simulink model "DYNctl_ver4_etud_obfusc"  (R2018b)
settings: Solver=ode45  StartTime=0.0  StopTime=tfin  FixedStep=0.001  RelTol=1e-9  AbsTol=1e-12  EnableMultiTasking=on
values from neighbouring files (symbols this model uses):
  denCompAngles = 1.0e07*[0.000000100000000 0.000823402569667 1.694979479335234 0]    [run_bancessai.m]
  denCompz = 1.0e05*[0.000010000000000 0.017380342819025 5.055406372627656 0]    [run_bancessai.m]
  g = sqrt(1+yp.^2)    [Trajectoire_func.m]
  numCompAngles = 1.0e09*[0.000230814504577 0.026170635469275 0.897433010674818 9.699372248008062]    [run_bancessai.m]
  numCompz = 1.0e11*[0.000031609546854 0.004304100455063 0.142047621936623 1.354942422178642]    [run_bancessai.m]
  TABC = [YA YB YC ... (first row only)    [run_bancessai.m]
  Tdef = [YD -XD 1 ... (first row only)    [run_bancessai.m]
undefined symbols (not defined in the file or in its folder): ae0, ae1, ae2, ae3, as0, as1, as2, as3, be1, JS, Jx, Jy, L, mS, mSg, mtot, R, rS, Vmax, XA, XB, XC, XD, XE, XF, YA, YB, YC, YD, YE, YF
settings Model: Creator=delafontaine  LastModifiedBy=natgo
settings SolverCC: AlgebraicLoopSolver=LineSearch
settings DataIOCC: LimitDataPoints=on  SaveFormat=Array  SignalLoggingSaveFormat=ModelDataLogs
settings OptimizationCC: LifeSpan=inf
settings DebuggingCC: UnderspecifiedInitializationDetection=Classic  MergeDetectMultiDrivingBlocksExec=none  MultiTaskDSMMsg=warning  MultiTaskCondExecSysMsg=none  SFUnexpectedBacktrackingDiag=warning  SFNoUnconditionalDefaultTransitionDiag=warning  SFExecutionAtInitializationDiag=none
settings HardwareCC: ProdBitPerPointer=32  ProdBitPerSizeT=32  ProdBitPerPtrDiffT=32  ProdLargestAtomicFloat=None  ProdIntDivRoundTo=Undefined  ProdEndianess=Unspecified  ProdWordSize=32  ProdHWDeviceType=32-bit Generic
settings ModelReferenceCC: PropagateSignalLabelsOutOfModel=off
settings SFSimCC: SimUseLocalCustomCode=off
settings RTWCC: RTWUseLocalCustomCode=off
settings CodeAppCC: StateflowObjectComments=on
settings GRTTargetCC: TargetLangStandard=C89/C90 (ANSI)  GeneratePreprocessorConditionals=Disable all
settings ConfigComp: CovMetricSettings=dw  CovHtmlReporting=on  CovSaveCumulativeToWorkspaceVar=on  CovSaveSingleToWorkspaceVar=on  CovExternalEMLEnable=off  CovSFcnEnable=off

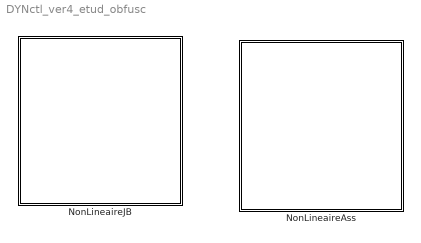
== system DYNctl_ver4_etud_obfusc ==
  NonLineaireAss : Subsystem
  NonLineaireJB : Subsystem

== system DYNctl_ver4_etud_obfusc/NonLineaireAss ==
  Asservissement 2 : Subsystem
  From Workspace1 : FromWorkspace  VariableName=z_des  SampleTime=0  Interpolate=off  OutputAfterFinalValue=Holding final value
  From Workspace4 : FromWorkspace  VariableName=x_des  SampleTime=0  Interpolate=off  OutputAfterFinalValue=Holding final value
  From Workspace6 : FromWorkspace  VariableName=y_des  SampleTime=0  Interpolate=off  OutputAfterFinalValue=Holding final value
  Mux1 : Mux  Inputs=25
  Systeme non lineaire : Subsystem
  To Workspace2 : ToWorkspace  VariableName=ySystemeNonLineaire  SampleTime=-1
  To Workspace6 : ToWorkspace  VariableName=Ax_des1  SampleTime=-1
  To Workspace7 : ToWorkspace  VariableName=Ay_des1  SampleTime=-1
  wires:
  Systeme non lineaire/6(Ib) -> Mux1/6
  Systeme non lineaire/21(zB) -> Mux1/21
  Systeme non lineaire/12(Wx) -> Mux1/12
  Asservissement 2/5(Vc) -> Systeme non lineaire/3(Vc)
  Asservissement 2/3(Va) -> Systeme non lineaire/1(Va)
  Asservissement 2/4(Vb) -> Systeme non lineaire/2(Vb)
  Systeme non lineaire/3(Vy) -> Asservissement 2/6(Vy), Mux1/3
  Systeme non lineaire/17(VA) -> Mux1/17
  Systeme non lineaire/23(zD) -> Asservissement 2/7(zD), Mux1/23
  Asservissement 2/1(Axcalcule) -> To Workspace6/1, Asservissement 2/11(Aydes)
  Systeme non lineaire/5(Ia) -> Mux1/5
  Systeme non lineaire/4(Vx) -> Asservissement 2/3(Vx), Mux1/4
  Systeme non lineaire/8(Ay) -> Mux1/8
  Systeme non lineaire/2(x) -> Asservissement 2/2(Px), Mux1/2
  Systeme non lineaire/9(Ax) -> Mux1/9
  Systeme non lineaire/15(Fb) -> Mux1/15
  Systeme non lineaire/16(Fc) -> Mux1/16
  Systeme non lineaire/1(y) -> Asservissement 2/5(Py), Mux1/1
  Systeme non lineaire/11(Vz) -> Mux1/11
  From Workspace4/1 -> Asservissement 2/1(xdes)
  Mux1/1 -> To Workspace2/1
  Systeme non lineaire/19(VC) -> Mux1/19
  Systeme non lineaire/13(Wy) -> Mux1/13
  Systeme non lineaire/7(Ic) -> Mux1/7
  Systeme non lineaire/10(Pz) -> Mux1/10
  Systeme non lineaire/22(zC) -> Mux1/22
  Asservissement 2/2(Aycalcule) -> To Workspace7/1, Asservissement 2/10(Axdes)
  Systeme non lineaire/25(zF) -> Asservissement 2/9(zF), Mux1/25
  Systeme non lineaire/20(zA) -> Mux1/20
  Systeme non lineaire/24(zE) -> Asservissement 2/8(zE), Mux1/24
  Systeme non lineaire/18(VB) -> Mux1/18
  Systeme non lineaire/14(Fa) -> Mux1/14
  From Workspace6/1 -> Asservissement 2/4(ydes)
  From Workspace1/1 -> Asservissement 2/12(zdes)

== system DYNctl_ver4_etud_obfusc/NonLineaireJB ==
  Asservissements : Subsystem
      mask help: Simulink:masks:GenSFuncDesc_MD
      mask Help: eval('feval(''rtwprivate'',''rtwhelpview'',''rtw_sfcn_block'')');
  Clock : Clock
  From Workspace2 : FromWorkspace  VariableName=x_des  SampleTime=0  Interpolate=off  OutputAfterFinalValue=Holding final value
  From Workspace3 : FromWorkspace  VariableName=y_des  SampleTime=0  Interpolate=off  OutputAfterFinalValue=Holding final value
  From Workspace5 : FromWorkspace  VariableName=z_des  SampleTime=0  Interpolate=off  OutputAfterFinalValue=Holding final value
  ModeleNonLineaire : Subsystem
      mask help: Simulink:masks:GenSFuncDesc_MD
      mask Help: eval('feval(''rtwprivate'',''rtwhelpview'',''rtw_sfcn_block'')');
  Mux : Mux  Inputs=25
  To Workspace : ToWorkspace  VariableName=tsim  SampleTime=-1
  To Workspace1 : ToWorkspace  VariableName=ynonlineaire  SampleTime=-1
  To Workspace10 : ToWorkspace  VariableName=z_des_out  SampleTime=-1
  To Workspace6 : ToWorkspace  VariableName=Ax_des  SampleTime=-1
  To Workspace7 : ToWorkspace  VariableName=Ay_des  SampleTime=-1
  To Workspace8 : ToWorkspace  VariableName=y_des_out  SampleTime=-1
  To Workspace9 : ToWorkspace  VariableName=x_des_out  SampleTime=-1
  wires:
  ModeleNonLineaire/7(Px) -> Asservissements/9(Px), Mux/7  "Px"
  ModeleNonLineaire/5(Wy) -> Mux/5  "Wy"
  From Workspace5/1 -> Asservissements/6(zdes), To Workspace10/1
  ModeleNonLineaire/18(zE) -> Asservissements/2(zE), Mux/18
  ModeleNonLineaire/1(Ax) -> Mux/1  "Ax"
  Asservissements/4(Axcalcule) -> Asservissements/4(Axdes), To Workspace6/1
  ModeleNonLineaire/11(IA) -> Mux/11  "IA"
  Clock/1 -> To Workspace/1
  ModeleNonLineaire/2(Ay) -> Mux/2  "Ay"
  Asservissements/5(Aycalcule) -> Asservissements/5(Aydes), To Workspace7/1
  ModeleNonLineaire/19(zF) -> Asservissements/3(zF), Mux/19
  Mux/1 -> To Workspace1/1
  ModeleNonLineaire/12(IB) -> Mux/12  "IB"
  ModeleNonLineaire/3(Pz) -> Mux/3  "Pz"
  ModeleNonLineaire/21(FB) -> Mux/21
  ModeleNonLineaire/17(zD) -> Asservissements/1(zD), Mux/17
  ModeleNonLineaire/24(VB) -> Mux/24
  ModeleNonLineaire/14(zA) -> Mux/14
  ModeleNonLineaire/9(Vx) -> Asservissements/11(Vx), Mux/9  "Vx"
  From Workspace2/1 -> Asservissements/7(xdes), To Workspace9/1
  ModeleNonLineaire/4(Wx) -> Mux/4  "Wx"
  ModeleNonLineaire/10(Vy) -> Asservissements/12(Vy), Mux/10  "Vy"
  ModeleNonLineaire/16(zC) -> Mux/16
  ModeleNonLineaire/15(zB) -> Mux/15
  ModeleNonLineaire/13(IC) -> Mux/13  "IC"
  ModeleNonLineaire/8(Py) -> Asservissements/10(Py), Mux/8  "Py"
  From Workspace3/1 -> Asservissements/8(ydes), To Workspace8/1
  ModeleNonLineaire/6(Vz) -> Mux/6  "Vz"
  ModeleNonLineaire/25(VC) -> Mux/25
  Asservissements/1(VAcalcule) -> ModeleNonLineaire/1(VAdesire)
  ModeleNonLineaire/22(FC) -> Mux/22
  Asservissements/3(VCcalcule) -> ModeleNonLineaire/3(VCdesire)
  ModeleNonLineaire/20(FA) -> Mux/20
  ModeleNonLineaire/23(VA) -> Mux/23
  Asservissements/2(VBcalcule) -> ModeleNonLineaire/2(VBdesire)

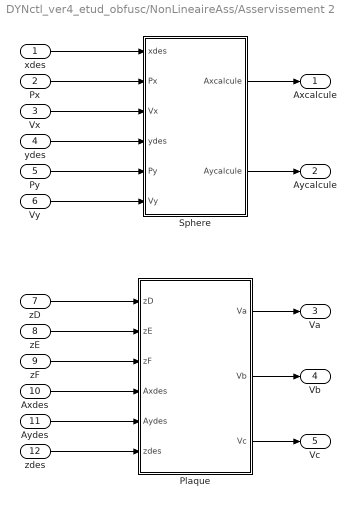
== system DYNctl_ver4_etud_obfusc/NonLineaireAss/Asservissement 2 ==
  xdes : Inport
  Px : Inport  Port=2
  Vx : Inport  Port=3
  ydes : Inport  Port=4
  Py : Inport  Port=5
  Vy : Inport  Port=6
  zD : Inport  Port=7
  zE : Inport  Port=8
  zF : Inport  Port=9
  Axdes : Inport  Port=10
  Aydes : Inport  Port=11
  zdes : Inport  Port=12
  Plaque : Subsystem
  Sphere : Subsystem
  Axcalcule : Outport
  Aycalcule : Outport  Port=2
  Va : Outport  Port=3
  Vb : Outport  Port=4
  Vc : Outport  Port=5
  wires:
  xdes/1 -> Sphere/1(xdes)
  Px/1 -> Sphere/2(Px)
  Vx/1 -> Sphere/3(Vx)
  ydes/1 -> Sphere/4(ydes)
  Py/1 -> Sphere/5(Py)
  Vy/1 -> Sphere/6(Vy)
  Sphere/1(Axcalcule) -> Axcalcule/1
  Sphere/2(Aycalcule) -> Aycalcule/1
  zD/1 -> Plaque/1(zD)
  zE/1 -> Plaque/2(zE)
  zF/1 -> Plaque/3(zF)
  Axdes/1 -> Plaque/4(Axdes)
  Aydes/1 -> Plaque/5(Aydes)
  zdes/1 -> Plaque/6(zdes)
  Plaque/1(Va) -> Va/1
  Plaque/2(Vb) -> Vb/1
  Plaque/3(Vc) -> Vc/1

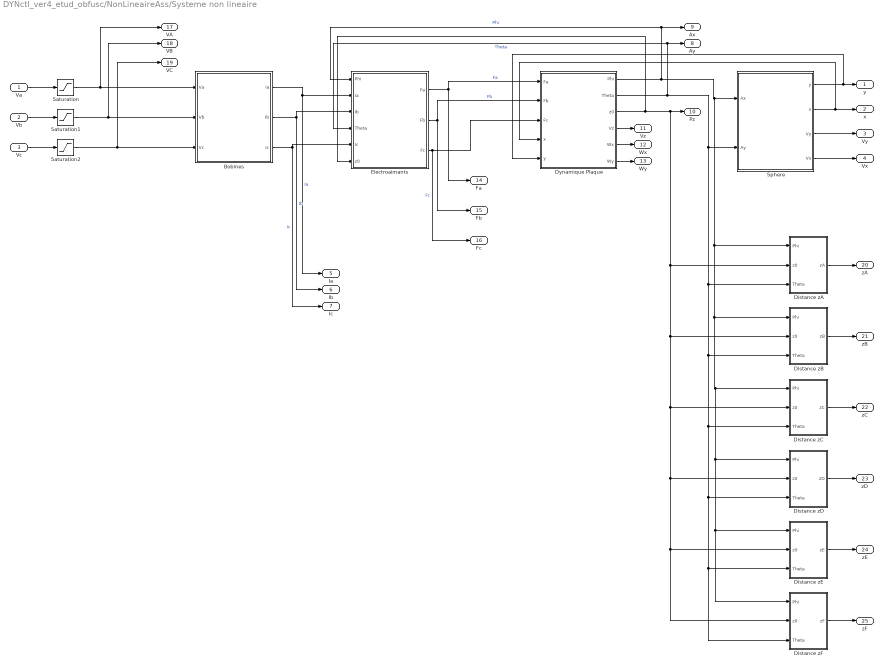
== system DYNctl_ver4_etud_obfusc/NonLineaireAss/Systeme non lineaire ==
  Va : Inport
  Vb : Inport  Port=2
  Vc : Inport  Port=3
  Bobines : Subsystem
  Distance zA : Subsystem
  Distance zB : Subsystem
  Distance zC : Subsystem
  Distance zD : Subsystem
  Distance zE : Subsystem
  Distance zF : Subsystem
  Dynamique Plaque : Subsystem
  Electroaimants : Subsystem
  Saturation : Saturate  UpperLimit=Vmax  LowerLimit=-Vmax
  Saturation1 : Saturate  UpperLimit=Vmax  LowerLimit=-Vmax
  Saturation2 : Saturate  UpperLimit=Vmax  LowerLimit=-Vmax
  Sphere : Subsystem
  y : Outport
  x : Outport  Port=2
  Vy : Outport  Port=3
  Vx : Outport  Port=4
  Ia : Outport  Port=5
  Ib : Outport  Port=6
  Ic : Outport  Port=7
  Ay : Outport  Port=8
  Ax : Outport  Port=9
  Pz : Outport  Port=10
  Vz : Outport  Port=11
  Wx : Outport  Port=12
  Wy : Outport  Port=13
  Fa : Outport  Port=14
  Fb : Outport  Port=15
  Fc : Outport  Port=16
  VA : Outport  Port=17
  VB : Outport  Port=18
  VC : Outport  Port=19
  zA : Outport  Port=20
  zB : Outport  Port=21
  zC : Outport  Port=22
  zD : Outport  Port=23
  zE : Outport  Port=24
  zF : Outport  Port=25
  wires:
  Bobines/2(Ib) -> Ib/1, Electroaimants/3(Ib)  "Ib"
  Bobines/1(Ia) -> Electroaimants/2(Ia), Ia/1  "Ia"
  Vb/1 -> Saturation1/1
  Va/1 -> Saturation/1
  Bobines/3(Ic) -> Ic/1, Electroaimants/5(Ic)  "Ic"
  Vc/1 -> Saturation2/1
  Sphere/1(y) -> y/1, Dynamique Plaque/5(y)
  Sphere/2(x) -> Dynamique Plaque/4(x), x/1
  Sphere/3(Vy) -> Vy/1
  Sphere/4(Vx) -> Vx/1
  Dynamique Plaque/4(Vz) -> Vz/1
  Dynamique Plaque/5(Wx) -> Wx/1
  Dynamique Plaque/6(Wy) -> Wy/1
  Saturation/1 -> Bobines/1(Va), VA/1
  Saturation2/1 -> Bobines/3(Vc), VC/1
  Saturation1/1 -> Bobines/2(Vb), VB/1
  Dynamique Plaque/3(z0) -> Distance zB/2(z0), Distance zF/2(z0), Distance zE/2(z0), Distance zD/2(z0), Distance zC/2(z0), Distance zA/2(z0), Pz/1, Electroaimants/6(z0)
  Distance zA/1(zA) -> zA/1
  Distance zB/1(zB) -> zB/1
  Distance zC/1(zC) -> zC/1
  Distance zD/1(zD) -> zD/1
  Distance zE/1(zE) -> zE/1
  Distance zF/1(zF) -> zF/1
  Electroaimants/1(Fa) -> Dynamique Plaque/1(Fa), Fa/1  "Fa"
  Electroaimants/2(Fb) -> Dynamique Plaque/2(Fb), Fb/1  "Fb"
  Electroaimants/3(Fc) -> Fc/1, Dynamique Plaque/3(Fc)  "Fc"
  Dynamique Plaque/1(Phi) -> Ax/1, Electroaimants/1(Phi), Distance zA/1(Phi), Distance zD/1(Phi), Distance zF/1(Phi), Distance zE/1(Phi), Distance zC/1(Phi), Distance zB/1(Phi), Sphere/1(Ax)  "Phi"
  Dynamique Plaque/2(Theta) -> Electroaimants/4(Theta), Ay/1, Distance zF/3(Theta), Distance zE/3(Theta), Distance zD/3(Theta), Distance zC/3(Theta), Distance zB/3(Theta), Distance zA/3(Theta), Sphere/2(Ay)  "Theta"

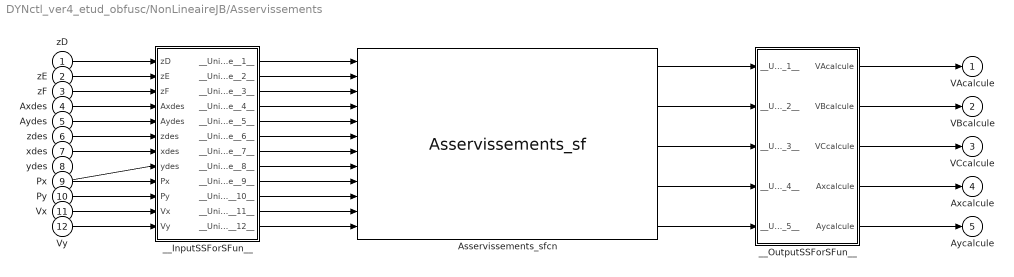
== system DYNctl_ver4_etud_obfusc/NonLineaireJB/Asservissements ==
  zD : Inport
  zE : Inport  Port=2
  zF : Inport  Port=3
  Axdes : Inport  Port=4
  Aydes : Inport  Port=5
  zdes : Inport  Port=6
  xdes : Inport  Port=7
  ydes : Inport  Port=8
  Px : Inport  Port=9
  Py : Inport  Port=10
  Vx : Inport  Port=11
  Vy : Inport  Port=12
  Asservissements_sfcn : S-Function  FunctionName=Asservissements_sf  SFunctionModules=""  SFunctionDeploymentMode=off  EnableBusSupport=off  mask{rtw_sf_name=Asservissements_sf, showVar=off}
      mask prompts: rtw_sf_name "Simulink:masks:GenSFuncName_MP"; showVar "Simulink:masks:GenSFuncShowModuleList_MP"
      mask help: Simulink:masks:GenSFuncDesc_MD
      mask init:
      | displist = '';
      | if ~strcmp(get_param(gcb, 'FunctionName'), rtw_sf_name);
      |   set_param(gcb, 'FunctionName', rtw_sf_name);
      | end
      | % Check if we are generating code
      | rtw_mode = false;
      | if strcmpi(get_param(bdroot(gcb),'SimulationStatus'),'Initializing')
      | 	rtw_mode = strcmpi(get_param(bdroot(gcb),'BuildingRTWCode'),'on') && ...
      | 		~strcmpi(get_param(bdroot(gcb),'TargetStyle'),'SimulationTarget');
      | end
      | if showVar || rtw_mode
      | 	if exist('rtwsfunc') == 2 | exist('rtwsfunc') == 6
      | 		tmplist = rtwsfunc(rtw_sf_name,gcb);
      | 		tmplist = DAStudio.message('Simulink:masks:GenSFuncListOfModules_IC', tmplist);
      | 	elseif showVar
      | 		tmplist1 = DAStudio.message('Simulink:masks:GenSFuncListOfModules_IC', '');
      |         tmplist2 = DAStudio.message('Simulink:masks:GenSFuncNotLicensed_IC');
      |         tmplist = [tmplist1 tmplist2];
      |  	end
      | end
      | if showVar
      |   displist = tmplist;
      | end
      settings: CopyFcn=|
      | if ~strcmp(get_param(gcb,'Linkstatus'),'none') && ...
      | ~strcmp(get_param(gcb,'Linkstatus'),'implicit')
      |   set_param(gcb,'LinkStatus','none');
      | end
      mask Help: eval('feval(''rtwprivate'',''rtwhelpview'',''rtw_sfcn_block'')');
      mask Display:
      | port_label('input',1,'zD');
      | port_label('input',2,'zE');
      | port_label('input',3,'zF');
      | port_label('input',4,'Axdes');
      | port_label('input',5,'Aydes');
      | port_label('input',6,'zdes');
      | port_label('input',7,'xdes');
      | port_label('input',8,'ydes');
      | port_label('input',9,'Px');
      | port_label('input',10,'Py');
      | port_label('input',11,'Vx');
      | port_label('input',12,'Vy');
      | port_label('output',1,'VAcalcule');
      | port_label('output',2,'VBcalcule');
      | port_label('output',3,'VCcalcule');
      | port_label('output',4,'Axcalcule');
      | port_label('output',5,'Aycalcule');
  __InputSSForSFun__ : Subsystem
  __OutputSSForSFun__ : Subsystem
  VAcalcule : Outport
  VBcalcule : Outport  Port=2
  VCcalcule : Outport  Port=3
  Axcalcule : Outport  Port=4
  Aycalcule : Outport  Port=5
  wires:
  zD/1 -> __InputSSForSFun__/1(zD)
  zE/1 -> __InputSSForSFun__/2(zE)
  zF/1 -> __InputSSForSFun__/3(zF)
  Axdes/1 -> __InputSSForSFun__/4(Axdes)
  Aydes/1 -> __InputSSForSFun__/5(Aydes)
  zdes/1 -> __InputSSForSFun__/6(zdes)
  xdes/1 -> __InputSSForSFun__/7(xdes)
  ydes/1 -> __InputSSForSFun__/8(ydes)
  Px/1 -> __InputSSForSFun__/9(Px)
  Py/1 -> __InputSSForSFun__/10(Py)
  Vx/1 -> __InputSSForSFun__/11(Vx)
  Vy/1 -> __InputSSForSFun__/12(Vy)
  __InputSSForSFun__/1(__UniqueOutportName__1__) -> Asservissements_sfcn/1
  __InputSSForSFun__/2(__UniqueOutportName__2__) -> Asservissements_sfcn/2
  __InputSSForSFun__/3(__UniqueOutportName__3__) -> Asservissements_sfcn/3
  __InputSSForSFun__/4(__UniqueOutportName__4__) -> Asservissements_sfcn/4
  __InputSSForSFun__/5(__UniqueOutportName__5__) -> Asservissements_sfcn/5
  __InputSSForSFun__/6(__UniqueOutportName__6__) -> Asservissements_sfcn/6
  __InputSSForSFun__/7(__UniqueOutportName__7__) -> Asservissements_sfcn/7
  __InputSSForSFun__/8(__UniqueOutportName__8__) -> Asservissements_sfcn/8
  __InputSSForSFun__/9(__UniqueOutportName__9__) -> Asservissements_sfcn/9
  __InputSSForSFun__/10(__UniqueOutportName__10__) -> Asservissements_sfcn/10
  __InputSSForSFun__/11(__UniqueOutportName__11__) -> Asservissements_sfcn/11
  __InputSSForSFun__/12(__UniqueOutportName__12__) -> Asservissements_sfcn/12
  Asservissements_sfcn/1 -> __OutputSSForSFun__/1(__UniqueInportName__1__)
  Asservissements_sfcn/2 -> __OutputSSForSFun__/2(__UniqueInportName__2__)
  Asservissements_sfcn/3 -> __OutputSSForSFun__/3(__UniqueInportName__3__)
  Asservissements_sfcn/4 -> __OutputSSForSFun__/4(__UniqueInportName__4__)
  Asservissements_sfcn/5 -> __OutputSSForSFun__/5(__UniqueInportName__5__)
  __OutputSSForSFun__/1(VAcalcule) -> VAcalcule/1
  __OutputSSForSFun__/2(VBcalcule) -> VBcalcule/1
  __OutputSSForSFun__/3(VCcalcule) -> VCcalcule/1
  __OutputSSForSFun__/4(Axcalcule) -> Axcalcule/1
  __OutputSSForSFun__/5(Aycalcule) -> Aycalcule/1

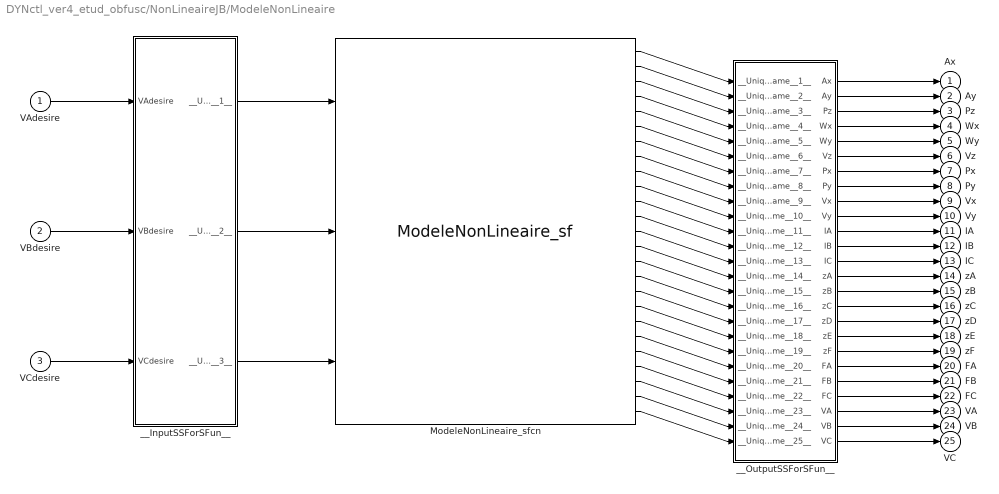
== system DYNctl_ver4_etud_obfusc/NonLineaireJB/ModeleNonLineaire ==
  VAdesire : Inport
  VBdesire : Inport  Port=2
  VCdesire : Inport  Port=3
  ModeleNonLineaire_sfcn : S-Function  FunctionName=ModeleNonLineaire_sf  SFunctionModules=""  SFunctionDeploymentMode=off  EnableBusSupport=off  mask{rtw_sf_name=ModeleNonLineaire_sf, showVar=off}
      mask prompts: rtw_sf_name "Simulink:masks:GenSFuncName_MP"; showVar "Simulink:masks:GenSFuncShowModuleList_MP"
      mask help: Simulink:masks:GenSFuncDesc_MD
      mask init: same as DYNctl_ver4_etud_obfusc/NonLineaireJB/Asservissements/Asservissements_sfcn
      settings: CopyFcn=|
      | if ~strcmp(get_param(gcb,'Linkstatus'),'none') && ...
      | ~strcmp(get_param(gcb,'Linkstatus'),'implicit')
      |   set_param(gcb,'LinkStatus','none');
      | end
      mask Help: eval('feval(''rtwprivate'',''rtwhelpview'',''rtw_sfcn_block'')');
      mask Display:
      | port_label('input',1,'VAdesire');
      | port_label('input',2,'VBdesire');
      | port_label('input',3,'VCdesire');
      | port_label('output',1,'Ax');
      | port_label('output',2,'Ay');
      | port_label('output',3,'Pz');
      | port_label('output',4,'Wx');
      | port_label('output',5,'Wy');
      | port_label('output',6,'Vz');
      | port_label('output',7,'Px');
      | port_label('output',8,'Py');
      | port_label('output',9,'Vx');
      | port_label('output',10,'Vy');
      | port_label('output',11,'IA');
      | port_label('output',12,'IB');
      | port_label('output',13,'IC');
      | port_label('output',14,'zA');
      | port_label('output',15,'zB');
      | port_label('output',16,'zC');
      | port_label('output',17,'zD');
      | port_label('output',18,'zE');
      | port_label('output',19,'zF');
      | port_label('output',20,'FA');
      | port_label('output',21,'FB');
      | port_label('output',22,'FC');
      | port_label('output',23,'VA');
      | port_label('output',24,'VB');
      | port_label('output',25,'VC');
  __InputSSForSFun__ : Subsystem
  __OutputSSForSFun__ : Subsystem
  Ax : Outport
  Ay : Outport  Port=2
  Pz : Outport  Port=3
  Wx : Outport  Port=4
  Wy : Outport  Port=5
  Vz : Outport  Port=6
  Px : Outport  Port=7
  Py : Outport  Port=8
  Vx : Outport  Port=9
  Vy : Outport  Port=10
  IA : Outport  Port=11
  IB : Outport  Port=12
  IC : Outport  Port=13
  zA : Outport  Port=14
  zB : Outport  Port=15
  zC : Outport  Port=16
  zD : Outport  Port=17
  zE : Outport  Port=18
  zF : Outport  Port=19
  FA : Outport  Port=20
  FB : Outport  Port=21
  FC : Outport  Port=22
  VA : Outport  Port=23
  VB : Outport  Port=24
  VC : Outport  Port=25
  wires:
  VAdesire/1 -> __InputSSForSFun__/1(VAdesire)
  VBdesire/1 -> __InputSSForSFun__/2(VBdesire)
  VCdesire/1 -> __InputSSForSFun__/3(VCdesire)
  __InputSSForSFun__/1(__UniqueOutportName__1__) -> ModeleNonLineaire_sfcn/1
  __InputSSForSFun__/2(__UniqueOutportName__2__) -> ModeleNonLineaire_sfcn/2
  __InputSSForSFun__/3(__UniqueOutportName__3__) -> ModeleNonLineaire_sfcn/3
  ModeleNonLineaire_sfcn/1 -> __OutputSSForSFun__/1(__UniqueInportName__1__)
  ModeleNonLineaire_sfcn/2 -> __OutputSSForSFun__/2(__UniqueInportName__2__)
  ModeleNonLineaire_sfcn/3 -> __OutputSSForSFun__/3(__UniqueInportName__3__)
  ModeleNonLineaire_sfcn/4 -> __OutputSSForSFun__/4(__UniqueInportName__4__)
  ModeleNonLineaire_sfcn/5 -> __OutputSSForSFun__/5(__UniqueInportName__5__)
  ModeleNonLineaire_sfcn/6 -> __OutputSSForSFun__/6(__UniqueInportName__6__)
  ModeleNonLineaire_sfcn/7 -> __OutputSSForSFun__/7(__UniqueInportName__7__)
  ModeleNonLineaire_sfcn/8 -> __OutputSSForSFun__/8(__UniqueInportName__8__)
  ModeleNonLineaire_sfcn/9 -> __OutputSSForSFun__/9(__UniqueInportName__9__)
  ModeleNonLineaire_sfcn/10 -> __OutputSSForSFun__/10(__UniqueInportName__10__)
  ModeleNonLineaire_sfcn/11 -> __OutputSSForSFun__/11(__UniqueInportName__11__)
  ModeleNonLineaire_sfcn/12 -> __OutputSSForSFun__/12(__UniqueInportName__12__)
  ModeleNonLineaire_sfcn/13 -> __OutputSSForSFun__/13(__UniqueInportName__13__)
  ModeleNonLineaire_sfcn/14 -> __OutputSSForSFun__/14(__UniqueInportName__14__)
  ModeleNonLineaire_sfcn/15 -> __OutputSSForSFun__/15(__UniqueInportName__15__)
  ModeleNonLineaire_sfcn/16 -> __OutputSSForSFun__/16(__UniqueInportName__16__)
  ModeleNonLineaire_sfcn/17 -> __OutputSSForSFun__/17(__UniqueInportName__17__)
  ModeleNonLineaire_sfcn/18 -> __OutputSSForSFun__/18(__UniqueInportName__18__)
  ModeleNonLineaire_sfcn/19 -> __OutputSSForSFun__/19(__UniqueInportName__19__)
  ModeleNonLineaire_sfcn/20 -> __OutputSSForSFun__/20(__UniqueInportName__20__)
  ModeleNonLineaire_sfcn/21 -> __OutputSSForSFun__/21(__UniqueInportName__21__)
  ModeleNonLineaire_sfcn/22 -> __OutputSSForSFun__/22(__UniqueInportName__22__)
  ModeleNonLineaire_sfcn/23 -> __OutputSSForSFun__/23(__UniqueInportName__23__)
  ModeleNonLineaire_sfcn/24 -> __OutputSSForSFun__/24(__UniqueInportName__24__)
  ModeleNonLineaire_sfcn/25 -> __OutputSSForSFun__/25(__UniqueInportName__25__)
  __OutputSSForSFun__/1(Ax) -> Ax/1
  __OutputSSForSFun__/2(Ay) -> Ay/1
  __OutputSSForSFun__/3(Pz) -> Pz/1
  __OutputSSForSFun__/4(Wx) -> Wx/1
  __OutputSSForSFun__/5(Wy) -> Wy/1
  __OutputSSForSFun__/6(Vz) -> Vz/1
  __OutputSSForSFun__/7(Px) -> Px/1
  __OutputSSForSFun__/8(Py) -> Py/1
  __OutputSSForSFun__/9(Vx) -> Vx/1
  __OutputSSForSFun__/10(Vy) -> Vy/1
  __OutputSSForSFun__/11(IA) -> IA/1
  __OutputSSForSFun__/12(IB) -> IB/1
  __OutputSSForSFun__/13(IC) -> IC/1
  __OutputSSForSFun__/14(zA) -> zA/1
  __OutputSSForSFun__/15(zB) -> zB/1
  __OutputSSForSFun__/16(zC) -> zC/1
  __OutputSSForSFun__/17(zD) -> zD/1
  __OutputSSForSFun__/18(zE) -> zE/1
  __OutputSSForSFun__/19(zF) -> zF/1
  __OutputSSForSFun__/20(FA) -> FA/1
  __OutputSSForSFun__/21(FB) -> FB/1
  __OutputSSForSFun__/22(FC) -> FC/1
  __OutputSSForSFun__/23(VA) -> VA/1
  __OutputSSForSFun__/24(VB) -> VB/1
  __OutputSSForSFun__/25(VC) -> VC/1

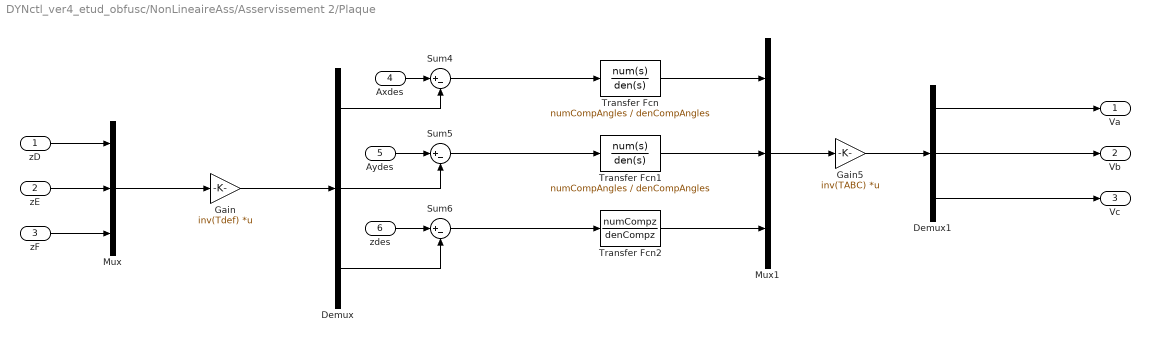
== system DYNctl_ver4_etud_obfusc/NonLineaireAss/Asservissement 2/Plaque ==
  zD : Inport
  zE : Inport  Port=2
  zF : Inport  Port=3
  Axdes : Inport  Port=4
  Aydes : Inport  Port=5
  zdes : Inport  Port=6
  Demux : Demux  Outputs=3
  Demux1 : Demux  Outputs=3
  Gain : Gain  Gain=inv(Tdef)  Multiplication=Matrix(K*u) (u vector)
  Gain5 : Gain  Gain=inv(TABC)  Multiplication=Matrix(K*u) (u vector)
  Mux : Mux  Inputs=3
  Mux1 : Mux  Inputs=3
  Sum4 : Sum  Inputs=|+-
  Sum5 : Sum  Inputs=|+-
  Sum6 : Sum  Inputs=|+-
  Transfer Fcn : TransferFcn  Numerator=numCompAngles  Denominator=denCompAngles
  Transfer Fcn1 : TransferFcn  Numerator=numCompAngles  Denominator=denCompAngles
  Transfer Fcn2 : TransferFcn  Numerator=numCompz  Denominator=denCompz
  Va : Outport
  Vb : Outport  Port=2
  Vc : Outport  Port=3
  wires:
  Axdes/1 -> Sum4/1
  Transfer Fcn2/1 -> Mux1/3
  zE/1 -> Mux/2
  Demux/1 -> Sum4/2
  Sum4/1 -> Transfer Fcn/1
  Mux/1 -> Gain/1
  Gain5/1 -> Demux1/1
  Mux1/1 -> Gain5/1
  Sum5/1 -> Transfer Fcn1/1
  Demux1/3 -> Vc/1
  zD/1 -> Mux/1
  zF/1 -> Mux/3
  Demux1/1 -> Va/1
  Sum6/1 -> Transfer Fcn2/1
  Demux1/2 -> Vb/1
  Gain/1 -> Demux/1
  Demux/2 -> Sum5/2
  Transfer Fcn/1 -> Mux1/1
  Aydes/1 -> Sum5/1
  Demux/3 -> Sum6/2
  Transfer Fcn1/1 -> Mux1/2
  zdes/1 -> Sum6/1

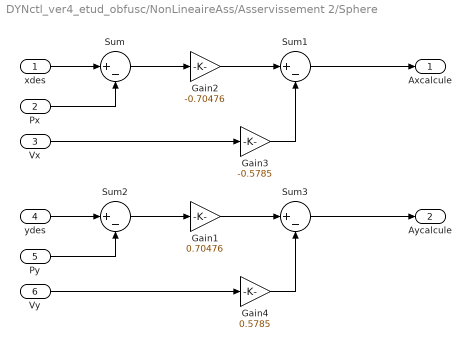
== system DYNctl_ver4_etud_obfusc/NonLineaireAss/Asservissement 2/Sphere ==
  xdes : Inport
  Px : Inport  Port=2
  Vx : Inport  Port=3
  ydes : Inport  Port=4
  Py : Inport  Port=5
  Vy : Inport  Port=6
  Gain1 : Gain  Gain=0.70476
  Gain2 : Gain  Gain=-0.70476
  Gain3 : Gain  Gain=-0.5785
  Gain4 : Gain  Gain=0.5785
  Sum{,1..3} (4 alike) : Sum  Inputs=|+-
  Axcalcule : Outport
  Aycalcule : Outport  Port=2
  wires:
  Py/1 -> Sum2/2
  Gain2/1 -> Sum1/1
  Sum2/1 -> Gain1/1
  Vx/1 -> Gain3/1
  ydes/1 -> Sum2/1
  Sum1/1 -> Axcalcule/1
  Sum/1 -> Gain2/1
  xdes/1 -> Sum/1
  Gain3/1 -> Sum1/2
  Vy/1 -> Gain4/1
  Gain1/1 -> Sum3/1
  Gain4/1 -> Sum3/2
  Sum3/1 -> Aycalcule/1
  Px/1 -> Sum/2

== system DYNctl_ver4_etud_obfusc/NonLineaireAss/Systeme non lineaire/Bobines ==
  Va : Inport
  Vb : Inport  Port=2
  Vc : Inport  Port=3
  Subsystem : Subsystem
  Subsystem1 : Subsystem
  Subsystem2 : Subsystem
  Ia : Outport
  Ib : Outport  Port=2
  Ic : Outport  Port=3
  wires:
  Va/1 -> Subsystem/1(In1)  "Va"
  Vb/1 -> Subsystem1/1(In1)  "Vb"
  Subsystem2/1(Out1) -> Ic/1  "Ic"
  Subsystem/1(Out1) -> Ia/1  "Ia"
  Vc/1 -> Subsystem2/1(In1)  "Vc"
  Subsystem1/1(Out1) -> Ib/1  "Ib"

== system DYNctl_ver4_etud_obfusc/NonLineaireAss/Systeme non lineaire/Distance zA ==
  Phi : Inport
  z0 : Inport  Port=2
  Theta : Inport  Port=3
  Gain : Gain  Gain=-XA
  Gain1 : Gain  Gain=YA
  Sum : Sum  Inputs=3
  zA : Outport
  wires:
  Sum/1 -> zA/1
  Gain/1 -> Sum/1
  Gain1/1 -> Sum/3
  z0/1 -> Sum/2
  Theta/1 -> Gain/1
  Phi/1 -> Gain1/1

== system DYNctl_ver4_etud_obfusc/NonLineaireAss/Systeme non lineaire/Distance zB ==
  Phi : Inport
  z0 : Inport  Port=2
  Theta : Inport  Port=3
  Gain : Gain  Gain=-XB
  Gain1 : Gain  Gain=YB
  Sum : Sum  Inputs=3
  zB : Outport
  wires:
  Sum/1 -> zB/1
  Gain/1 -> Sum/1
  Gain1/1 -> Sum/3
  z0/1 -> Sum/2
  Theta/1 -> Gain/1
  Phi/1 -> Gain1/1

== system DYNctl_ver4_etud_obfusc/NonLineaireAss/Systeme non lineaire/Distance zC ==
  Phi : Inport
  z0 : Inport  Port=2
  Theta : Inport  Port=3
  Gain : Gain  Gain=-XC
  Gain1 : Gain  Gain=YC
  Sum : Sum  Inputs=3
  zC : Outport
  wires:
  Sum/1 -> zC/1
  Gain/1 -> Sum/1
  Gain1/1 -> Sum/3
  z0/1 -> Sum/2
  Theta/1 -> Gain/1
  Phi/1 -> Gain1/1

== system DYNctl_ver4_etud_obfusc/NonLineaireAss/Systeme non lineaire/Distance zD ==
  Phi : Inport
  z0 : Inport  Port=2
  Theta : Inport  Port=3
  Gain : Gain  Gain=-XD
  Gain1 : Gain  Gain=YD
  Sum : Sum  Inputs=3
  zD : Outport
  wires:
  Sum/1 -> zD/1
  Gain/1 -> Sum/1
  Gain1/1 -> Sum/3
  z0/1 -> Sum/2
  Phi/1 -> Gain1/1
  Theta/1 -> Gain/1

== system DYNctl_ver4_etud_obfusc/NonLineaireAss/Systeme non lineaire/Distance zE ==
  Phi : Inport
  z0 : Inport  Port=2
  Theta : Inport  Port=3
  Gain : Gain  Gain=-XE
  Gain1 : Gain  Gain=YE
  Sum : Sum  Inputs=3
  zE : Outport
  wires:
  Sum/1 -> zE/1
  Gain/1 -> Sum/1
  Gain1/1 -> Sum/3
  z0/1 -> Sum/2
  Theta/1 -> Gain/1
  Phi/1 -> Gain1/1

== system DYNctl_ver4_etud_obfusc/NonLineaireAss/Systeme non lineaire/Distance zF ==
  Phi : Inport
  z0 : Inport  Port=2
  Theta : Inport  Port=3
  Gain : Gain  Gain=-XF
  Gain1 : Gain  Gain=YF
  Sum : Sum  Inputs=3
  zF : Outport
  wires:
  Sum/1 -> zF/1
  Gain/1 -> Sum/1
  Gain1/1 -> Sum/3
  z0/1 -> Sum/2
  Theta/1 -> Gain/1
  Phi/1 -> Gain1/1

== system DYNctl_ver4_etud_obfusc/NonLineaireAss/Systeme non lineaire/Dynamique Plaque ==
  Fa : Inport
  Fb : Inport  Port=2
  Fc : Inport  Port=3
  x : Inport  Port=4
  y : Inport  Port=5
  Subsystem : Subsystem
  Subsystem1 : Subsystem
  Subsystem2 : Subsystem
  Phi : Outport
  Theta : Outport  Port=2
  z0 : Outport  Port=3
  Vz : Outport  Port=4
  Wx : Outport  Port=5
  Wy : Outport  Port=6
  wires:
  Fa/1 -> Subsystem1/3(In3), Subsystem2/2(In2)  "Fa"
  Fc/1 -> Subsystem/2(In2), Subsystem1/2(In2), Subsystem2/3(In3)  "Fc"
  Subsystem1/1(Theta) -> Theta/1
  Fb/1 -> Subsystem1/1(In1), Subsystem/1(In1), Subsystem2/1(In1)  "Fb"
  Subsystem/1(Phi) -> Phi/1
  Subsystem2/1(z0) -> z0/1
  Subsystem2/2(Vz) -> Vz/1
  Subsystem/2(Wx) -> Wx/1
  Subsystem1/2(Wy) -> Wy/1
  x/1 -> Subsystem1/4(x)
  y/1 -> Subsystem/3(y)

== system DYNctl_ver4_etud_obfusc/NonLineaireAss/Systeme non lineaire/Electroaimants ==
  Phi : Inport
  Ia : Inport  Port=2
  Ib : Inport  Port=3
  Theta : Inport  Port=4
  Ic : Inport  Port=5
  z0 : Inport  Port=6
  Subsystem : Subsystem
  Subsystem1 : Subsystem
  Subsystem2 : Subsystem
  Fa : Outport
  Fb : Outport  Port=2
  Fc : Outport  Port=3
  wires:
  z0/1 -> Subsystem2/4(In4), Subsystem1/4(In4), Subsystem/4(In4)  "z0"
  Theta/1 -> Subsystem2/3(In3), Subsystem/3(In3), Subsystem1/3(In3)  "Theta"
  Ic/1 -> Subsystem2/1(In1)  "Ic"
  Phi/1 -> Subsystem/2(In2), Subsystem2/2(In2), Subsystem1/2(In2)  "Phi"
  Subsystem2/1(Out1) -> Fc/1  "Fc"
  Ia/1 -> Subsystem/1(In1)  "Ia"
  Ib/1 -> Subsystem1/1(In1)  "Ib"
  Subsystem1/1(Out1) -> Fb/1  "Fb"
  Subsystem/1(Out1) -> Fa/1  "Fa"

== system DYNctl_ver4_etud_obfusc/NonLineaireAss/Systeme non lineaire/Sphere ==
  Ax : Inport
  Ay : Inport  Port=2
  Gain : Gain
  Subsystem3 : Subsystem
  Subsystem4 : Subsystem
  y : Outport
  x : Outport  Port=2
  Vy : Outport  Port=3
  Vx : Outport  Port=4
  wires:
  Subsystem3/2(Out1) -> Vy/1  "Vy"
  Subsystem4/1(Out4) -> x/1  "x"
  Subsystem3/1(Out4) -> y/1  "y"
  Ay/1 -> Gain/1
  Subsystem4/2(Out1) -> Vx/1  "Vx"
  Gain/1 -> Subsystem4/1(In4)
  Ax/1 -> Subsystem3/1(In4)  "Phi"

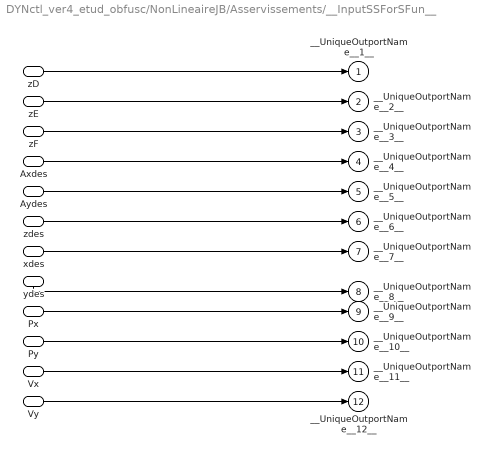
== system DYNctl_ver4_etud_obfusc/NonLineaireJB/Asservissements/__InputSSForSFun__ ==
  zD : Inport
  zE : Inport  Port=2
  zF : Inport  Port=3
  Axdes : Inport  Port=4
  Aydes : Inport  Port=5
  zdes : Inport  Port=6
  xdes : Inport  Port=7
  ydes : Inport  Port=8
  Px : Inport  Port=9
  Py : Inport  Port=10
  Vx : Inport  Port=11
  Vy : Inport  Port=12
  __UniqueOutportName__1__ : Outport
  __UniqueOutportName__2__ : Outport  Port=2
  __UniqueOutportName__3__ : Outport  Port=3
  __UniqueOutportName__4__ : Outport  Port=4
  __UniqueOutportName__5__ : Outport  Port=5
  __UniqueOutportName__6__ : Outport  Port=6
  __UniqueOutportName__7__ : Outport  Port=7
  __UniqueOutportName__8__ : Outport  Port=8
  __UniqueOutportName__9__ : Outport  Port=9
  __UniqueOutportName__10__ : Outport  Port=10
  __UniqueOutportName__11__ : Outport  Port=11
  __UniqueOutportName__12__ : Outport  Port=12
  wires:
  zD/1 -> __UniqueOutportName__1__/1
  zE/1 -> __UniqueOutportName__2__/1
  zF/1 -> __UniqueOutportName__3__/1
  Axdes/1 -> __UniqueOutportName__4__/1
  Aydes/1 -> __UniqueOutportName__5__/1
  zdes/1 -> __UniqueOutportName__6__/1
  xdes/1 -> __UniqueOutportName__7__/1
  ydes/1 -> __UniqueOutportName__8__/1
  Px/1 -> __UniqueOutportName__9__/1
  Py/1 -> __UniqueOutportName__10__/1
  Vx/1 -> __UniqueOutportName__11__/1
  Vy/1 -> __UniqueOutportName__12__/1

== system DYNctl_ver4_etud_obfusc/NonLineaireJB/Asservissements/__OutputSSForSFun__ ==
  __UniqueInportName__1__ : Inport
  __UniqueInportName__2__ : Inport  Port=2
  __UniqueInportName__3__ : Inport  Port=3
  __UniqueInportName__4__ : Inport  Port=4
  __UniqueInportName__5__ : Inport  Port=5
  VAcalcule : Outport
  VBcalcule : Outport  Port=2
  VCcalcule : Outport  Port=3
  Axcalcule : Outport  Port=4
  Aycalcule : Outport  Port=5
  wires:
  __UniqueInportName__1__/1 -> VAcalcule/1
  __UniqueInportName__2__/1 -> VBcalcule/1
  __UniqueInportName__3__/1 -> VCcalcule/1
  __UniqueInportName__4__/1 -> Axcalcule/1  "Ax_des"
  __UniqueInportName__5__/1 -> Aycalcule/1  "Ay_des"

== system DYNctl_ver4_etud_obfusc/NonLineaireJB/ModeleNonLineaire/__InputSSForSFun__ ==
  VAdesire : Inport
  VBdesire : Inport  Port=2
  VCdesire : Inport  Port=3
  __UniqueOutportName__1__ : Outport
  __UniqueOutportName__2__ : Outport  Port=2
  __UniqueOutportName__3__ : Outport  Port=3
  wires:
  VAdesire/1 -> __UniqueOutportName__1__/1
  VBdesire/1 -> __UniqueOutportName__2__/1
  VCdesire/1 -> __UniqueOutportName__3__/1

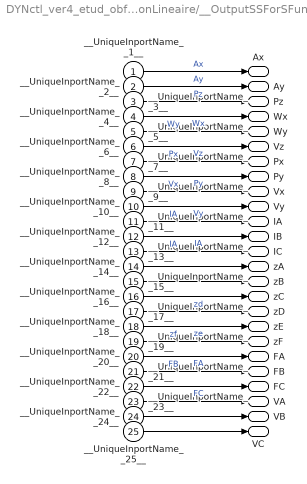
== system DYNctl_ver4_etud_obfusc/NonLineaireJB/ModeleNonLineaire/__OutputSSForSFun__ ==
  __UniqueInportName__1__ : Inport
  __UniqueInportName__2__ : Inport  Port=2
  __UniqueInportName__3__ : Inport  Port=3
  __UniqueInportName__4__ : Inport  Port=4
  __UniqueInportName__5__ : Inport  Port=5
  __UniqueInportName__6__ : Inport  Port=6
  __UniqueInportName__7__ : Inport  Port=7
  __UniqueInportName__8__ : Inport  Port=8
  __UniqueInportName__9__ : Inport  Port=9
  __UniqueInportName__10__ : Inport  Port=10
  __UniqueInportName__11__ : Inport  Port=11
  __UniqueInportName__12__ : Inport  Port=12
  __UniqueInportName__13__ : Inport  Port=13
  __UniqueInportName__14__ : Inport  Port=14
  __UniqueInportName__15__ : Inport  Port=15
  __UniqueInportName__16__ : Inport  Port=16
  __UniqueInportName__17__ : Inport  Port=17
  __UniqueInportName__18__ : Inport  Port=18
  __UniqueInportName__19__ : Inport  Port=19
  __UniqueInportName__20__ : Inport  Port=20
  __UniqueInportName__21__ : Inport  Port=21
  __UniqueInportName__22__ : Inport  Port=22
  __UniqueInportName__23__ : Inport  Port=23
  __UniqueInportName__24__ : Inport  Port=24
  __UniqueInportName__25__ : Inport  Port=25
  Ax : Outport
  Ay : Outport  Port=2
  Pz : Outport  Port=3
  Wx : Outport  Port=4
  Wy : Outport  Port=5
  Vz : Outport  Port=6
  Px : Outport  Port=7
  Py : Outport  Port=8
  Vx : Outport  Port=9
  Vy : Outport  Port=10
  IA : Outport  Port=11
  IB : Outport  Port=12
  IC : Outport  Port=13
  zA : Outport  Port=14
  zB : Outport  Port=15
  zC : Outport  Port=16
  zD : Outport  Port=17
  zE : Outport  Port=18
  zF : Outport  Port=19
  FA : Outport  Port=20
  FB : Outport  Port=21
  FC : Outport  Port=22
  VA : Outport  Port=23
  VB : Outport  Port=24
  VC : Outport  Port=25
  wires:
  __UniqueInportName__1__/1 -> Ax/1  "Ax"
  __UniqueInportName__2__/1 -> Ay/1  "Ay"
  __UniqueInportName__3__/1 -> Pz/1  "Pz"
  __UniqueInportName__4__/1 -> Wx/1  "Wx"
  __UniqueInportName__5__/1 -> Wy/1  "Wy"
  __UniqueInportName__6__/1 -> Vz/1  "Vz"
  __UniqueInportName__7__/1 -> Px/1  "Px"
  __UniqueInportName__8__/1 -> Py/1  "Py"
  __UniqueInportName__9__/1 -> Vx/1  "Vx"
  __UniqueInportName__10__/1 -> Vy/1  "Vy"
  __UniqueInportName__11__/1 -> IA/1  "IA"
  __UniqueInportName__12__/1 -> IB/1  "IA"
  __UniqueInportName__13__/1 -> IC/1  "IA"
  __UniqueInportName__14__/1 -> zA/1
  __UniqueInportName__15__/1 -> zB/1
  __UniqueInportName__16__/1 -> zC/1
  __UniqueInportName__17__/1 -> zD/1  "zd"
  __UniqueInportName__18__/1 -> zE/1  "ze"
  __UniqueInportName__19__/1 -> zF/1  "zf"
  __UniqueInportName__20__/1 -> FA/1  "FA"
  __UniqueInportName__21__/1 -> FB/1  "FB"
  __UniqueInportName__22__/1 -> FC/1  "FC"
  __UniqueInportName__23__/1 -> VA/1
  __UniqueInportName__24__/1 -> VB/1
  __UniqueInportName__25__/1 -> VC/1

== system DYNctl_ver4_etud_obfusc/NonLineaireAss/Systeme non lineaire/Bobines/Subsystem ==
  note: Ia
  note: Va
  In1 : Inport
  Gain : Gain  Gain=1/L
  Gain1 : Gain  Gain=R/L
  Integrator : Integrator
  Sum : Sum  Inputs=|+-
  Out1 : Outport
  wires:
  Integrator/1 -> Out1/1, Gain1/1
  Gain/1 -> Sum/1
  Gain1/1 -> Sum/2
  Sum/1 -> Integrator/1
  In1/1 -> Gain/1

== system DYNctl_ver4_etud_obfusc/NonLineaireAss/Systeme non lineaire/Bobines/Subsystem1 ==
  In1 : Inport
  Gain : Gain  Gain=1/L
  Gain1 : Gain  Gain=R/L
  Integrator : Integrator
  Sum : Sum  Inputs=|+-
  Out1 : Outport
  wires:
  Integrator/1 -> Out1/1, Gain1/1
  Gain/1 -> Sum/1
  Gain1/1 -> Sum/2
  Sum/1 -> Integrator/1
  In1/1 -> Gain/1

== system DYNctl_ver4_etud_obfusc/NonLineaireAss/Systeme non lineaire/Bobines/Subsystem2 ==
  In1 : Inport
  Gain : Gain  Gain=1/L
  Gain1 : Gain  Gain=R/L
  Integrator : Integrator
  Sum : Sum  Inputs=|+-
  Out1 : Outport
  wires:
  Integrator/1 -> Out1/1, Gain1/1
  Gain/1 -> Sum/1
  Gain1/1 -> Sum/2
  Sum/1 -> Integrator/1
  In1/1 -> Gain/1

== system DYNctl_ver4_etud_obfusc/NonLineaireAss/Systeme non lineaire/Dynamique Plaque/Subsystem ==
  In1 : Inport
  In2 : Inport  Port=2
  y : Inport  Port=3
  Gain : Gain  Gain=mSg
  Gain10 : Gain  Gain=YB
  Gain11 : Gain  Gain=YC
  Gain12 : Gain  Gain=1/Jx
  Integrator : Integrator
  Integrator1 : Integrator
  Sum9 : Sum  Inputs=|+++
  Phi : Outport
  Wx : Outport  Port=2
  wires:
  Integrator1/1 -> Phi/1
  In2/1 -> Gain11/1
  Integrator/1 -> Wx/1, Integrator1/1
  Gain10/1 -> Sum9/1
  Sum9/1 -> Gain12/1
  Gain12/1 -> Integrator/1
  Gain11/1 -> Sum9/2
  In1/1 -> Gain10/1
  Gain/1 -> Sum9/3
  y/1 -> Gain/1

== system DYNctl_ver4_etud_obfusc/NonLineaireAss/Systeme non lineaire/Dynamique Plaque/Subsystem1 ==
  note: Fa
  note: Fc
  note: Fb
  In1 : Inport
  In2 : Inport  Port=2
  In3 : Inport  Port=3
  x : Inport  Port=4
  Gain : Gain  Gain=mSg
  Gain13 : Gain  Gain=XB
  Gain14 : Gain  Gain=XC
  Gain15 : Gain  Gain=1/Jy
  Gain16 : Gain  Gain=XA
  Integrator1 : Integrator
  Integrator2 : Integrator
  Sum10 : Sum  Inputs=|----
  Theta : Outport
  Wy : Outport  Port=2
  wires:
  In3/1 -> Gain16/1
  Gain14/1 -> Sum10/2
  Gain15/1 -> Integrator2/1
  Sum10/1 -> Gain15/1
  In1/1 -> Gain13/1
  Gain13/1 -> Sum10/1
  Integrator2/1 -> Wy/1, Integrator1/1
  In2/1 -> Gain14/1
  Gain16/1 -> Sum10/3
  Integrator1/1 -> Theta/1
  x/1 -> Gain/1
  Gain/1 -> Sum10/4

== system DYNctl_ver4_etud_obfusc/NonLineaireAss/Systeme non lineaire/Dynamique Plaque/Subsystem2 ==
  note: Fc
  note: Fa
  note: Fb
  In1 : Inport
  In2 : Inport  Port=2
  In3 : Inport  Port=3
  Constant : Constant  Value=g
  Gain17 : Gain  Gain=1/mtot
  Integrator4 : Integrator
  Integrator5 : Integrator  InitialCondition=0.015
  Sum : Sum  Inputs=|++
  Sum11 : Sum  Inputs=|+++
  z0 : Outport
  Vz : Outport  Port=2
  wires:
  Integrator5/1 -> z0/1  "z0"
  In3/1 -> Sum11/3
  Sum11/1 -> Gain17/1
  In1/1 -> Sum11/2
  Integrator4/1 -> Vz/1, Integrator5/1
  Gain17/1 -> Sum/1
  In2/1 -> Sum11/1
  Sum/1 -> Integrator4/1
  Constant/1 -> Sum/2

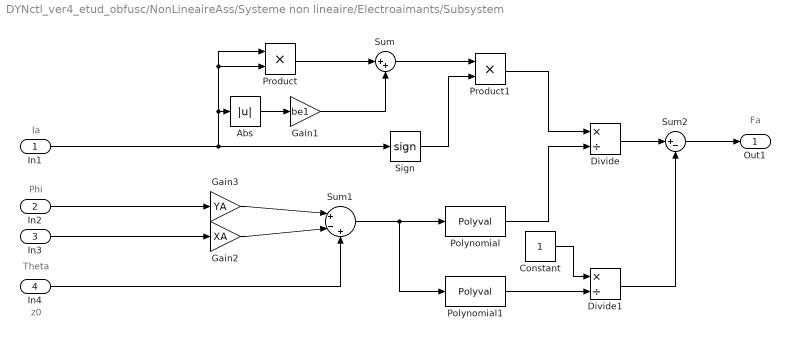
== system DYNctl_ver4_etud_obfusc/NonLineaireAss/Systeme non lineaire/Electroaimants/Subsystem ==
  note: Fa
  note: z0
  note: Theta
  note: Phi
  note: Ia
  In1 : Inport
  In2 : Inport  Port=2
  In3 : Inport  Port=3
  In4 : Inport  Port=4
  Abs : Abs
  Constant : Constant
  Divide : Product  Inputs=*/
  Divide1 : Product  Inputs=*/
  Gain1 : Gain  Gain=be1
  Gain2 : Gain  Gain=XA
  Gain3 : Gain  Gain=YA
  Polynomial : Polyval  Coefs=[ae3 ae2 ae1 ae0]
  Polynomial1 : Polyval  Coefs=[as3 as2 as1 as0]
  Product : Product
  Product1 : Product
  Sign : Signum
  Sum : Sum  Inputs=|++
  Sum1 : Sum  Inputs=|+-+
  Sum2 : Sum  Inputs=|+-
  Out1 : Outport
  wires:
  Sum/1 -> Product1/1
  Product1/1 -> Divide/1
  Gain2/1 -> Sum1/2
  Sum2/1 -> Out1/1
  Constant/1 -> Divide1/1
  Product/1 -> Sum/1
  Polynomial/1 -> Divide/2
  In1/1 -> Product/1, Product/2, Abs/1, Sign/1
  Abs/1 -> Gain1/1
  Gain1/1 -> Sum/2
  Polynomial1/1 -> Divide1/2
  Sum1/1 -> Polynomial1/1, Polynomial/1
  Sign/1 -> Product1/2
  In4/1 -> Sum1/3
  Divide/1 -> Sum2/1
  Gain3/1 -> Sum1/1
  Divide1/1 -> Sum2/2
  In2/1 -> Gain3/1
  In3/1 -> Gain2/1

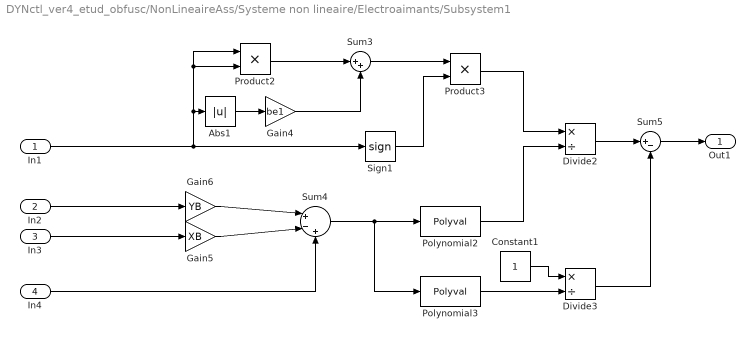
== system DYNctl_ver4_etud_obfusc/NonLineaireAss/Systeme non lineaire/Electroaimants/Subsystem1 ==
  In1 : Inport
  In2 : Inport  Port=2
  In3 : Inport  Port=3
  In4 : Inport  Port=4
  Abs1 : Abs
  Constant1 : Constant
  Divide2 : Product  Inputs=*/
  Divide3 : Product  Inputs=*/
  Gain4 : Gain  Gain=be1
  Gain5 : Gain  Gain=XB
  Gain6 : Gain  Gain=YB
  Polynomial2 : Polyval  Coefs=[ae3 ae2 ae1 ae0]
  Polynomial3 : Polyval  Coefs=[as3 as2 as1 as0]
  Product2 : Product
  Product3 : Product
  Sign1 : Signum
  Sum3 : Sum  Inputs=|++
  Sum4 : Sum  Inputs=|+-+
  Sum5 : Sum  Inputs=|+-
  Out1 : Outport
  wires:
  In2/1 -> Gain6/1
  Gain6/1 -> Sum4/1
  In4/1 -> Sum4/3
  Gain5/1 -> Sum4/2
  Sum4/1 -> Polynomial3/1, Polynomial2/1
  In1/1 -> Product2/1, Product2/2, Abs1/1, Sign1/1
  Constant1/1 -> Divide3/1
  Sign1/1 -> Product3/2
  Divide2/1 -> Sum5/1
  In3/1 -> Gain5/1
  Divide3/1 -> Sum5/2
  Polynomial3/1 -> Divide3/2
  Product3/1 -> Divide2/1
  Gain4/1 -> Sum3/2
  Abs1/1 -> Gain4/1
  Product2/1 -> Sum3/1
  Sum3/1 -> Product3/1
  Polynomial2/1 -> Divide2/2
  Sum5/1 -> Out1/1

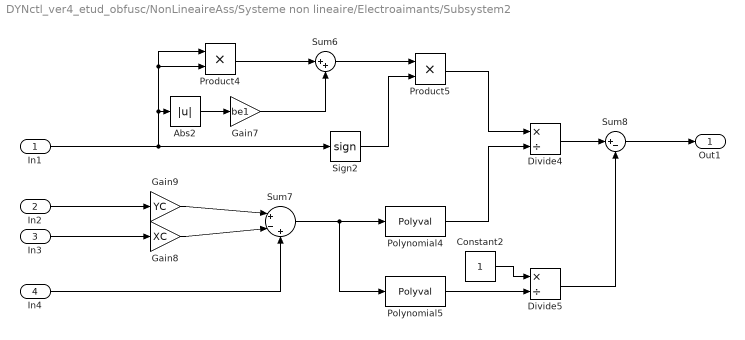
== system DYNctl_ver4_etud_obfusc/NonLineaireAss/Systeme non lineaire/Electroaimants/Subsystem2 ==
  In1 : Inport
  In2 : Inport  Port=2
  In3 : Inport  Port=3
  In4 : Inport  Port=4
  Abs2 : Abs
  Constant2 : Constant
  Divide4 : Product  Inputs=*/
  Divide5 : Product  Inputs=*/
  Gain7 : Gain  Gain=be1
  Gain8 : Gain  Gain=XC
  Gain9 : Gain  Gain=YC
  Polynomial4 : Polyval  Coefs=[ae3 ae2 ae1 ae0]
  Polynomial5 : Polyval  Coefs=[as3 as2 as1 as0]
  Product4 : Product
  Product5 : Product
  Sign2 : Signum
  Sum6 : Sum  Inputs=|++
  Sum7 : Sum  Inputs=|+-+
  Sum8 : Sum  Inputs=|+-
  Out1 : Outport
  wires:
  Gain9/1 -> Sum7/1
  Gain8/1 -> Sum7/2
  Divide5/1 -> Sum8/2
  Divide4/1 -> Sum8/1
  Constant2/1 -> Divide5/1
  In1/1 -> Product4/1, Product4/2, Abs2/1, Sign2/1
  Sum7/1 -> Polynomial5/1, Polynomial4/1
  Sign2/1 -> Product5/2
  In2/1 -> Gain9/1
  Product4/1 -> Sum6/1
  Product5/1 -> Divide4/1
  In4/1 -> Sum7/3
  Polynomial5/1 -> Divide5/2
  Gain7/1 -> Sum6/2
  Polynomial4/1 -> Divide4/2
  Sum6/1 -> Product5/1
  Abs2/1 -> Gain7/1
  Sum8/1 -> Out1/1
  In3/1 -> Gain8/1

== system DYNctl_ver4_etud_obfusc/NonLineaireAss/Systeme non lineaire/Sphere/Subsystem3 ==
  note: y
  note: Vy
  note: Phi
  In4 : Inport  Tag=Theta
  Gain : Gain  Gain=mS*g/(mS+JS/rS^2)
  Integrator : Integrator
  Integrator1 : Integrator
  Out4 : Outport
  Out1 : Outport  Port=2
  wires:
  Gain/1 -> Integrator/1
  In4/1 -> Gain/1
  Integrator1/1 -> Out4/1
  Integrator/1 -> Out1/1, Integrator1/1

== system DYNctl_ver4_etud_obfusc/NonLineaireAss/Systeme non lineaire/Sphere/Subsystem4 ==
  In4 : Inport  Tag=Theta
  Gain : Gain  Gain=-mS*g/(mS+JS/rS^2)
  Integrator : Integrator
  Integrator1 : Integrator
  Out4 : Outport
  Out1 : Outport  Port=2
  wires:
  Gain/1 -> Integrator/1
  In4/1 -> Gain/1
  Integrator1/1 -> Out4/1
  Integrator/1 -> Out1/1, Integrator1/1
